simulink model "Outer1NoActions"  (Simulink 9.0)
settings: Solver=ode45  StartTime=0.0  StopTime=10.0  RelTol=1e-3  EnableMultiTasking=on
settings Model: SuppressorTable=22 serialization::archive 11 0 6 0 0 0 0 0  Creator=scaife  LastModifiedBy=ktrinh  ExtModeAutoUpdateStatusClock=off
settings DataIOCC: LimitDataPoints=on  SignalLoggingSaveFormat=ModelDataLogs  SignalLoggingName=sigsOut
settings DebuggingCC: SaveWithParameterizedLinksMsg=none  SignalResolutionControl=TryResolveAllWithWarning  MultiTaskDSMMsg=warning  MultiTaskCondExecSysMsg=none
settings HardwareCC: TargetUnknown=on
settings SFSimCC: SimParseCustomCode=off
settings GRTTargetCC: CombineOutputUpdateFcns=off  GRTInterface=on

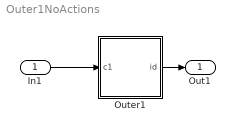
== system Outer1NoActions ==
  In1 : Inport  OutDataTypeStr=boolean
  Outer1 : Stateflow chart  TreatAsAtomicUnit=on
  Out1 : Outport
  wires:
  Outer1/1(id) -> Out1/1
  In1/1 -> Outer1/1(c1)

== stateflow chart Outer1 ==
  state A/
    en: id=1;
  A -> A : [c1]
  (default) -> A
  data: c1 input double; id output double
